simulink model "PFC_by_VFD_IM"  (R2024a)
settings: Solver=VariableStepAuto  StartTime=0.0  StopTime=2  RelTol=1e-3
libraries: spsRMSLib x2, spsUniversalBridgeLib x2, spsAsynchronousMachineSIUnitsLib x1, spsPower3phInstantaneousLib x1, spsSeriesRLCBranchLib x1, spsThreePhaseVIMeasurementLib x1, spsThreePhaseSourceLib x1, sps_lib x1
settings Model: Creator=User  LastModifiedBy=User
settings SolverCC: ZeroCrossAlgorithm=Adaptive
settings DebuggingCC: IgnoredZcDiagnostic=none

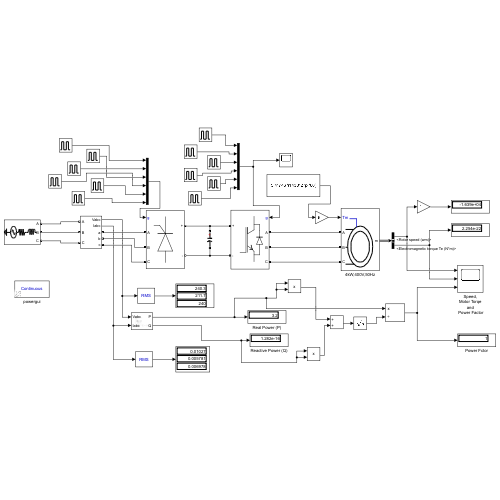
[thumbnail: Simulink's stored preview of the top-level diagram]
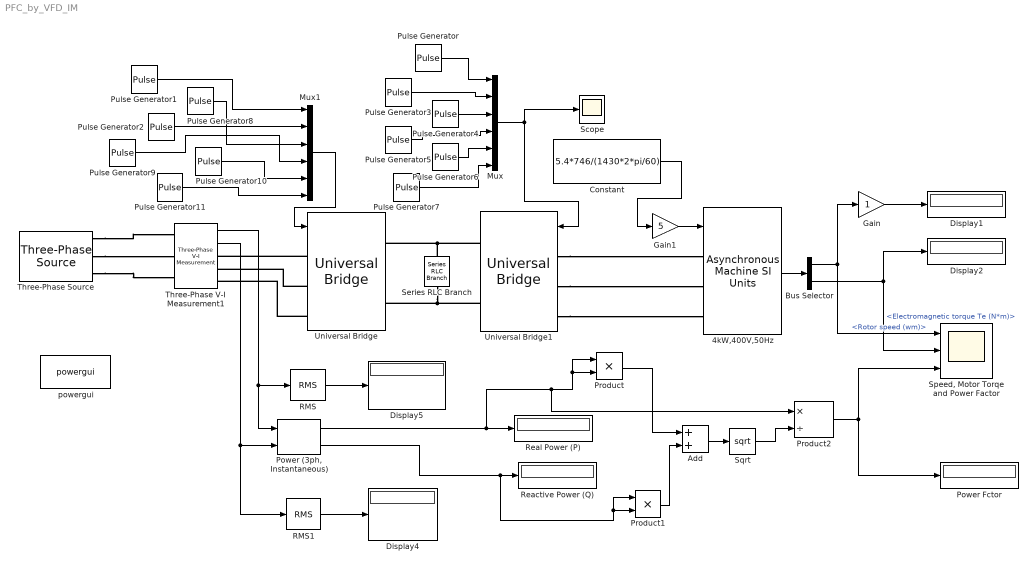
== system PFC_by_VFD_IM ==
  4kW,400V,50Hz : spsAsynchronousMachineSIUnitsLib/Asynchronous Machine SI Units  RotorType=Squirrel-cage  PresetModel="15:  5.4 HP (4KW)   400 V  50Hz 1430 RPM"  MechanicalLoad=Torque Tm  ShowDetailedParameters=on  ReferenceFrame=Rotor  Units=SI  MeasurementBus=off  NominalParameters=[4000 400 50]  VoltageRatio=1  Stator=[1.405 0.005839]  Rotor=[1.395 0.005839]  Cage1=[0.4155 0.002066]  Cage2=[0.4168 0.0003495]  Lm=0.1722  Mechanical=[0.0131 0.002985 2]  PolePairs=2  InitialConditions=[0 0 0 0 0 0 0 0]  SimulateSaturation=off  Saturation=[14.03593122, 27.81365428, 53.79336849, 72.68890987, 97.98006896, 148.6815601, 215.7428561, 302.9841135, 428.7778367 ; 230, 322, 414, 460, 506, 552, 598, 644, 690]  LoadFlowParameters=1492000  TsPowergui=0  TsBlock=-1  IterativeModel=Trapezoidal non iterative  IterativeDiscreteModel=Trapezoidal non iterative  Pmec=1.492e+006
  Add : Sum
  Bus Selector : BusSelector  OutputSignals=Mechanical.Rotor speed (wm),Mechanical.Electromagnetic torque Te (N*m)
  Constant : Constant  Value=5.4*746/(1430*2*pi/60)
  Display{1..2,4..5} (4 alike) : Display
  Gain : Gain
  Gain1 : Gain  Gain=5
  Mux : Mux  Inputs=6
  Mux1 : Mux  Inputs=6
  "Power (3ph, Instantaneous)" : spsPower3phInstantaneousLib/Power (3ph, Instantaneous)
  Power Fctor : Display
  Product : Product
  Product1 : Product
  Product2 : Product  Inputs=*/
  Pulse Generator : DiscretePulseGenerator  PulseType=Time based  Period=0.05  PulseWidth=50  PhaseDelay=0.05/6
  Pulse Generator1 : DiscretePulseGenerator  PulseType=Time based  Period=1/50  PulseWidth=6.667e-3
  Pulse Generator10 : DiscretePulseGenerator  PulseType=Time based  Period=1/50  PulseWidth=6.667e-3  PhaseDelay=240
  Pulse Generator11 : DiscretePulseGenerator  PulseType=Time based  Period=1/50  PulseWidth=6.667e-3  PhaseDelay=300
  Pulse Generator2 : DiscretePulseGenerator  PulseType=Time based  Period=1/50  PulseWidth=6.667e-3  PhaseDelay=60
  Pulse Generator3 : DiscretePulseGenerator  PulseType=Time based  Period=0.05  PulseWidth=50  PhaseDelay=2*(0.05/6)
  Pulse Generator4 : DiscretePulseGenerator  PulseType=Time based  Period=0.05  PulseWidth=50  PhaseDelay=3*(0.05/6)
  Pulse Generator5 : DiscretePulseGenerator  PulseType=Time based  Period=0.05  PulseWidth=50  PhaseDelay=4*(0.05/6)
  Pulse Generator6 : DiscretePulseGenerator  PulseType=Time based  Period=0.05  PulseWidth=50  PhaseDelay=5*(0.05/6)
  Pulse Generator7 : DiscretePulseGenerator  PulseType=Time based  Period=0.05  PulseWidth=50  PhaseDelay=6*(0.05/6)
  Pulse Generator8 : DiscretePulseGenerator  PulseType=Time based  Period=1/50  PulseWidth=6.667e-3  PhaseDelay=120
  Pulse Generator9 : DiscretePulseGenerator  PulseType=Time based  Period=1/50  PulseWidth=6.667e-3  PhaseDelay=180
  RMS : spsRMSLib/RMS  TrueRMS=on  Freq=60  RMSInit=120  Ts=0
  RMS1 : spsRMSLib/RMS  TrueRMS=on  Freq=60  RMSInit=120  Ts=0
  Reactive Power (Q) : Display
  Real Power (P) : Display
  Scope : Scope
  Series RLC Branch : spsSeriesRLCBranchLib/Series RLC Branch  LConnTagsString=__new0  RConnTagsString=__new0  BranchType=C  Resistance=1  Inductance=1e-3  SetiL0=off  InitialCurrent=0  Capacitance=1e-6  Setx0=off  InitialVoltage=0  Measurements=None
  "Speed, Motor Torqe and Power Factor" : Scope  NumInputPorts=3
  Sqrt : Sqrt
  Three-Phase V-I Measurement1 : spsThreePhaseVIMeasurementLib/Three-Phase V-I Measurement  VoltageMeasurement=phase-to-ground  SetLabelV=off  LabelV=Vabc  Vpu=off  VpuLL=off  CurrentMeasurement=yes  SetLabelI=off  LabelI=Iabc  Ipu=off  Pbase=100e6  Vbase=500e3  OutputType=Complex  PhasorSimulation=off  PSBequivalent=0
  Three-Phase Source : spsThreePhaseSourceLib/Three-Phase Source  InternalConnection=Yg  VoltagePhases=off  Voltage=400  PhaseAngle=0  Voltage_phases=[25e3 25e3 25e3]/sqrt(3)  PhaseAngles_phases=[0 -120 +120]  Frequency=50  NonIdealSource=on  SpecifyImpedance=off  Resistance=0.8929  Inductance=16.58e-3  ShortCircuitLevel=100e6  BaseVoltage=400  XRratio=7  BusType=swing  Pref=10e3  Qref=0  Prefabc=[10e3, 10e3, 10e3]  Qrefabc=[0, 0, 0]  Qmin=-inf  Qmax=inf
  Universal Bridge : spsUniversalBridgeLib/Universal Bridge  Arms=3  SnubberResistance=1e5  SnubberCapacitance=inf  Device=Thyristors  Ron=1e-3  Lon=0  ForwardVoltages="[  0  0  ]"  ForwardVoltage=0  GTOparameters=[ 10e-6 , 20e-6 ]  IGBTparameters=[ 1e-6 , 2e-6 ]  Measurements=None  Measurements_2=None  converterType=Rectifier
  Universal Bridge1 : spsUniversalBridgeLib/Universal Bridge  Arms=3  SnubberResistance=1e5  SnubberCapacitance=inf  Device=IGBT / Diodes  Ron=1e-3  Lon=0  ForwardVoltages="[  0  0  ]"  ForwardVoltage=0  GTOparameters=[ 10e-6 , 20e-6 ]  IGBTparameters=[ 1e-6 , 2e-6 ]  Measurements=None  Measurements_2=None  converterType=Rectifier
  powergui : sps_lib/powergui  Priority=1  SimulationMode=Continuous  SampleTime=50e-6  frequency=60  Iterations=50  frequencyindice=50  Pbase=100e6  ErrMax=1e-4  UnitsV=kV  UnitsW=MW  buscounter=0  FunctionMessages=off  echomessages=off  EnableUseOfTLC=off  CurrentSourceSwitches=off  DisableSnubberDevices=off  DisableRonSwitches=off  DisableVfSwitches=off  DisplayEquations=off  AutomaticDiscreteSolvers=off  SolverType=Tustin/Backward Euler (TBE)  Interpol=off  ExternalGateDelay=off  methode=off  Ts=100  x0status=blocks  SPID=on  SwTol=0  HookPort=off  NonlinearTolerance=1e-4  nMaxIteration=100  ContinueOnMaxIteration=off  RestoreLinks=warning  ResistiveCurrentMeasurement=off  Frange=[0:2:500]  Ylog=off  Xlog=on  ShowGrid=off  save=off  variable=ZData  structure=0  ZoomFFT=off  StartTime=0.0  cycles=1  DisplayStyle=1  fundamental=60  FreqAxis=off  MaxFrequency=1000  frequencyindicesteady=1  RmsSteady=1  display=off
  wires:
  Three-Phase V-I Measurement1/1 -> "Power (3ph, Instantaneous)"/1, RMS/1
  Three-Phase V-I Measurement1/2 -> "Power (3ph, Instantaneous)"/2, RMS1/1
  Add/1 -> Sqrt/1
  "Power (3ph, Instantaneous)"/2 -> Product1/2, Product1/1, Reactive Power (Q)/1
  Product2/1 -> "Speed, Motor Torqe and Power Factor"/3, Power Fctor/1
  Product/1 -> Add/1
  Product1/1 -> Add/2
  Gain/1 -> Display1/1
  Gain1/1 -> 4kW,400V,50Hz/1
  4kW,400V,50Hz/1 -> Bus Selector/1
  RMS/1 -> Display5/1
  Sqrt/1 -> Product2/2
  Bus Selector/1 -> Gain/1, "Speed, Motor Torqe and Power Factor"/1  "<Rotor speed (wm)>"
  Bus Selector/2 -> Display2/1, "Speed, Motor Torqe and Power Factor"/2  "<Electromagnetic torque Te (N*m)>"
  RMS1/1 -> Display4/1
  "Power (3ph, Instantaneous)"/1 -> Product2/1, Product/2, Product/1, Real Power (P)/1
  Constant/1 -> Gain1/1
  Mux/1 -> Scope/1, Universal Bridge1/1
  Pulse Generator/1 -> Mux/1
  Pulse Generator3/1 -> Mux/2
  Pulse Generator4/1 -> Mux/3
  Pulse Generator5/1 -> Mux/4
  Pulse Generator6/1 -> Mux/5
  Pulse Generator7/1 -> Mux/6
  Pulse Generator2/1 -> Mux1/2
  Pulse Generator1/1 -> Mux1/1
  Pulse Generator8/1 -> Mux1/3
  Pulse Generator9/1 -> Mux1/4
  Pulse Generator10/1 -> Mux1/5
  Pulse Generator11/1 -> Mux1/6
  Mux1/1 -> Universal Bridge/1
  connections:
  Three-Phase Source/RConn3 -- Three-Phase V-I Measurement1/LConn3
  Three-Phase Source/RConn2 -- Three-Phase V-I Measurement1/LConn2
  Three-Phase Source/RConn1 -- Three-Phase V-I Measurement1/LConn1
  Universal Bridge/LConn1 -- Three-Phase V-I Measurement1/RConn1
  Universal Bridge/LConn2 -- Three-Phase V-I Measurement1/RConn2
  Universal Bridge/LConn3 -- Three-Phase V-I Measurement1/RConn3
  Series RLC Branch/LConn1 -- Universal Bridge/RConn1 -- Universal Bridge1/RConn1
  Series RLC Branch/RConn1 -- Universal Bridge1/RConn2 -- Universal Bridge/RConn2
  Universal Bridge1/LConn1 -- 4kW,400V,50Hz/LConn1
  Universal Bridge1/LConn2 -- 4kW,400V,50Hz/LConn2
  Universal Bridge1/LConn3 -- 4kW,400V,50Hz/LConn3
